simulink model "sldemo_foreach_vectorized"  (Simulink 7.6)
settings: Solver=FixedStepDiscrete  StartTime=0.0  StopTime=1.0  RelTol=1e-3
libraries: simulink x1
settings Model: Creator=The MathWorks Inc.
settings DataIOCC: SaveFormat=Structure
settings OptimizationCC: OptimizeModelRefInitCode=on  LifeSpan=1
settings RTWCC: SystemTargetFile=ert.tlc  TemplateMakefile=ert_default_tmf  Description=Real-Time Workshop Embedded Coder  GenerateReport=on  ProcessScript=ert_make_rtw_hook  IncludeHyperlinkInReport=on  LaunchReport=on
settings CodeAppCC: IgnoreCustomStorageClasses=off
settings ERTTargetCC: MultiwordLength=2048  GenerateSampleERTMain=on  MatFileLogging=on  SupportVariableSizeSignals=on  ERTCustomFileTemplate=example_file_process.tlc  ConvertIfToSwitch=off

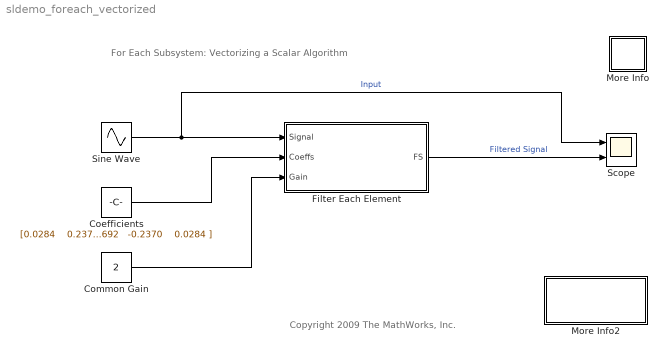
== system sldemo_foreach_vectorized ==
  note: Copyright 2009 The MathWorks, Inc.
  note: For Each Subsystem:
      | Vectorizing a Scalar Algorithm
  Coefficients : Constant  Value=|
      | [0.0284    0.2370    0.4692    0.2370    0.0284
      | ;   -0.0651   -0.0000    0.8698   -0.0000   -0.0651
      |  ;   0.0284   -0.2370    0.4692   -0.2370    0.0284
      | ]
  Common Gain : Constant  Value=2
  Filter Each Element : Subsystem  TreatAsAtomicUnit=on
      settings: RTWFcnNameOpts=Use subsystem name  RTWFileNameOpts=Use function name
  More Info : Subsystem
      settings: OpenFcn=showdemo(bdroot(gcb))
      mask Display: disp('?')
  More Info2 : Subsystem
      settings: OpenFcn=sldemo_foreach_repeat_scalar
      mask Display: disp('Double-Click for\nNon Vectorized\nImplementation')
  Scope : Scope  NumInputPorts=2
      settings: YMin=-5~-5  YMax=5~5
  Sine Wave : Sin  Amplitude=[1 1 1]  Frequency=[25 15 5]*pi  SampleTime=1/30
  wires:
  Sine Wave/1 -> Filter Each Element/1(Signal), Scope/1  "Input"
  Coefficients/1 -> Filter Each Element/2(Coeffs)
  Common Gain/1 -> Filter Each Element/3(Gain)
  Filter Each Element/1(FS) -> Scope/2  "Filtered Signal"

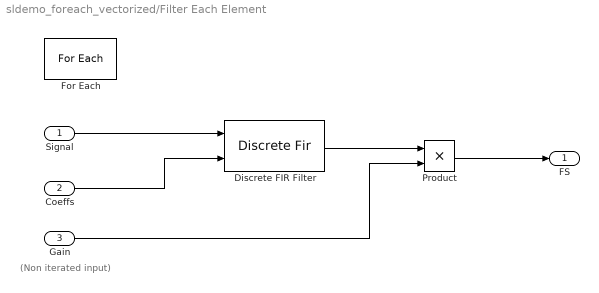
== system sldemo_foreach_vectorized/Filter Each Element ==
  note: (Non iterated input)
  Signal : Inport  Partition=on  PartitionDimension=1  PartitionWidth=1
  Coeffs : Inport  Port=2  Partition=on  PartitionDimension=1  PartitionWidth=1
  Gain : Inport  Port=3  Partition=off
  Discrete FIR Filter : DiscreteFir  CoefSource=Input port
  For Each : ForEach  IndexMode=One-based
  Product : Product  RndMeth=Zero
  FS : Outport  ConcatenationDimension=1
  wires:
  Coeffs/1 -> Discrete FIR Filter/2
  Signal/1 -> Discrete FIR Filter/1
  Discrete FIR Filter/1 -> Product/1
  Gain/1 -> Product/2
  Product/1 -> FS/1

== system sldemo_foreach_vectorized/More Info ==
  note: Bus Block Demonstration
  note: This demonstration shows how signals may be grouped and ungrouped while
      | retaining their names.  In this demonstration, 5 signals are created and labeled
      | appropriately.  These signals are then mux'd together to create a bus of signals.
      | This bus of signals is then fed into the Bus Selector block.  Inside of the Bus
      | Selector block, the Pulse and Chirp signals are chosen to be output from the
      | original signal bus.
      |
      | It is possible to place a nest signal buses and then still retrieve the original signal
      | with its label.

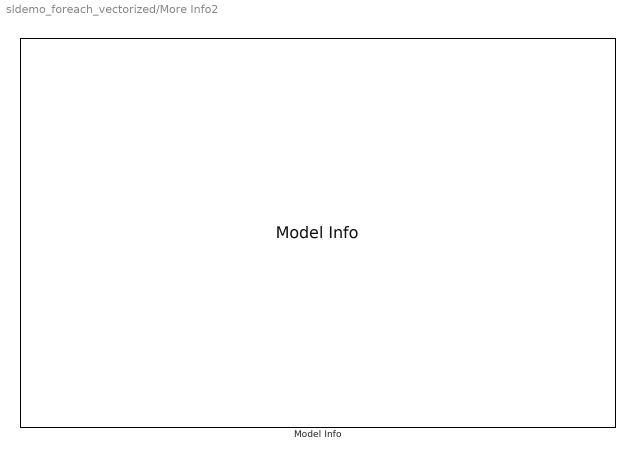
== system sldemo_foreach_vectorized/More Info2 ==
  Model Info : simulink/Model-Wide Utilities/Model Info  SystemSampleTime=-1  InitialBlockCM=None  BlockCM=none  Frame=on  DisplayStringWithTags=Model Info  HorizontalTextAlignment=Left  LeftAlignmentValue=0.02  SourceBlockDiagram=sldemo_foreach_vectorized  TagMaxNumber=20
